simulink model "PAA"  (R2018b)
settings: Solver=FixedStepAuto  StartTime=0.0  StopTime=t_sim  RelTol=1e-3
values from neighbouring files (symbols this model uses):
  FLAG_INPUT_SIGNAL = 0    [PAA_evaluation.m]    (also in door.m)
  noise_gain = 0    [PAA_evaluation.m]    (also in door.m)
  plant_denominator_spr_parallel = [1, -0.1, 0.64]    [PAA_evaluation.m]    (also in door.m)
  t_AdapOff = t_sim+1    (= 4)    [PAA_evaluation.m]    (also in door.m = 5)
  t_AdapOn = 0    [PAA_evaluation.m]    (also in door.m)
  Ts = 0.01    [PAA_evaluation.m]    (also in door.m)
undefined symbols (not defined in the file or in its folder): adap_init
libraries: simulink x3
settings Model: Creator=litingsun  LastModifiedBy=jessl
settings SFSimCC: SimUseLocalCustomCode=off
settings RTWCC: RTWUseLocalCustomCode=off
settings CodeAppCC: StateflowObjectComments=on

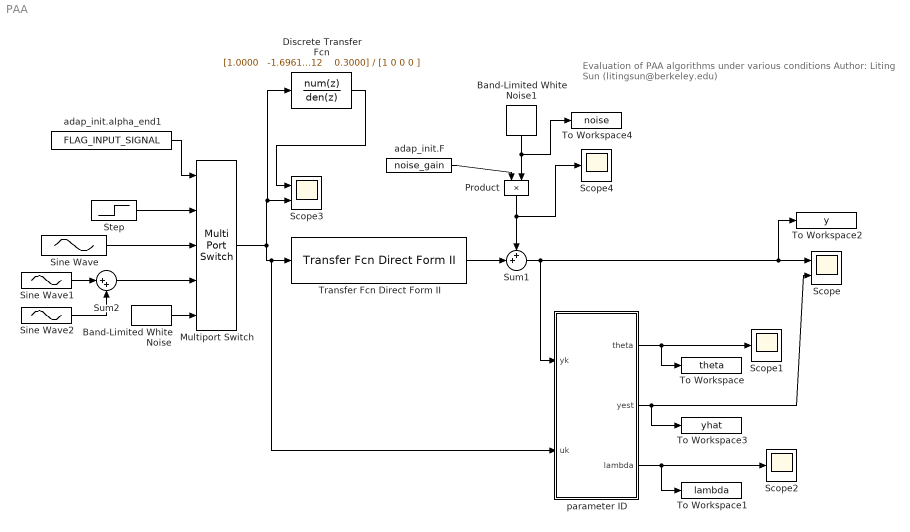
== system PAA ==
  note: Evaluation of PAA algorithms under various conditions
      |
      | Author: Liting Sun (litingsun@berkeley.edu)
  Band-Limited White Noise : simulink/Sources/Band-Limited White Noise  Cov=[0.1]  Ts=Ts  seed=[23341]
  Band-Limited White Noise1 : simulink/Sources/Band-Limited White Noise  Cov=[1]  Ts=Ts  seed=[12345]
  Discrete Transfer Fcn : DiscreteTransferFcn  Numerator="[1.0000   -1.6961    0.4012    0.3000]"  Denominator=[1 0 0 0 ]
  Multiport Switch : MultiPortSwitch  DataPortOrder=Zero-based contiguous  Inputs=4  zeroidx=on
  Product : Product
  Scope : Scope  NumInputPorts=2
  Scope1 : Scope
  Scope2 : Scope
  Scope3 : Scope  NumInputPorts=2
  Scope4 : Scope
  Sine Wave : Sin  Amplitude=0.1  Frequency=2*pi  SampleTime=0
  Sine Wave1 : Sin  Amplitude=1.1  Frequency=10  SampleTime=0
  Sine Wave2 : Sin  Amplitude=2.7  Frequency=97  SampleTime=0
  Step : Step  SampleTime=Ts
  Sum1 : Sum  Inputs=++|
  Sum2 : Sum  Inputs=|++
  To Workspace : ToWorkspace  VariableName=theta  SaveFormat=Structure With Time  SampleTime=-1
  To Workspace1 : ToWorkspace  VariableName=lambda  SaveFormat=Structure With Time  SampleTime=-1
  To Workspace2 : ToWorkspace  VariableName=y  SaveFormat=Structure With Time  SampleTime=-1
  To Workspace3 : ToWorkspace  VariableName=yhat  SaveFormat=Structure With Time  SampleTime=-1
  To Workspace4 : ToWorkspace  VariableName=noise  SaveFormat=Structure With Time  SampleTime=-1
  Transfer Fcn Direct Form II : simulink/Additional Math & Discrete/Additional Discrete/Transfer Fcn Direct Form II  NumCoefVec=[0, 2, 1]  DenCoefVec=plant_denominator_spr_parallel(2:3)  vinit=0.0  RndMeth=Zero  DoSatur=off
      settings: SourceProductName=Simulink  SourceProductBaseCode=SL
  "adap_init.F " : Constant  Value=noise_gain
  adap_init.alpha_end1 : Constant  Value=FLAG_INPUT_SIGNAL
  parameter ID : Subsystem
  wires:
  parameter ID/1(theta) -> Scope1/1, To Workspace/1
  parameter ID/3(lambda) -> Scope2/1, To Workspace1/1
  parameter ID/2(yest) -> Scope/2, To Workspace3/1
  Multiport Switch/1 -> Discrete Transfer Fcn/1, Scope3/2, parameter ID/2(uk), Transfer Fcn Direct Form II/1
  Transfer Fcn Direct Form II/1 -> Sum1/2
  Band-Limited White Noise1/1 -> To Workspace4/1, Product/2
  Product/1 -> Scope4/1, Sum1/1
  "adap_init.F "/1 -> Product/1
  Sum1/1 -> Scope/1, To Workspace2/1, parameter ID/1(yk)
  adap_init.alpha_end1/1 -> Multiport Switch/1
  Step/1 -> Multiport Switch/2
  Band-Limited White Noise/1 -> Multiport Switch/5
  Sine Wave/1 -> Multiport Switch/3
  Sine Wave1/1 -> Sum2/1
  Sine Wave2/1 -> Sum2/2
  Sum2/1 -> Multiport Switch/4
  Discrete Transfer Fcn/1 -> Scope3/1

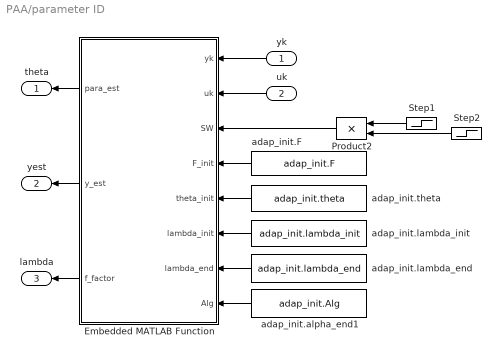
== system PAA/parameter ID ==
  yk : Inport
  uk : Inport  Port=2
  Embedded MATLAB Function : MATLAB Function  TreatAsAtomicUnit=on
  Product2 : Product  RndMeth=Zero
  Step1 : Step  Time=t_AdapOn  SampleTime=Ts
  Step2 : Step  Time=t_AdapOff  Before=1  After=0  SampleTime=Ts
  "adap_init.F " : Constant  Value=adap_init.F
  adap_init.alpha_end1 : Constant  Value=adap_init.Alg
  adap_init.lambda_end : Constant  Value=adap_init.lambda_end
  adap_init.lambda_init : Constant  Value=adap_init.lambda_init
  adap_init.theta : Constant  Value=adap_init.theta
  theta : Outport
  yest : Outport  Port=2
  lambda : Outport  Port=3
  wires:
  uk/1 -> Embedded MATLAB Function/2(uk)
  Embedded MATLAB Function/3(f_factor) -> lambda/1
  "adap_init.F "/1 -> Embedded MATLAB Function/4(F_init)
  adap_init.alpha_end1/1 -> Embedded MATLAB Function/8(Alg)
  Embedded MATLAB Function/1(para_est) -> theta/1
  adap_init.lambda_init/1 -> Embedded MATLAB Function/6(lambda_init)
  yk/1 -> Embedded MATLAB Function/1(yk)
  adap_init.lambda_end/1 -> Embedded MATLAB Function/7(lambda_end)
  Product2/1 -> Embedded MATLAB Function/3(SW)
  Step2/1 -> Product2/2
  Step1/1 -> Product2/1
  adap_init.theta/1 -> Embedded MATLAB Function/5(theta_init)
  Embedded MATLAB Function/2(y_est) -> yest/1

== matlab function PAA/parameter ID/Embedded MATLAB Function ==
  data: yk input; uk input; SW input; para_est output; y_est output; f_factor output; F_init input; theta_init input; lambda_init input; lambda_end input; Alg input
function [para_est, y_est, f_factor] = PAA(yk,uk, SW, F_init,theta_init,lambda_init,lambda_end, Alg) %#eml
persistent N y u phi F theta lambda yhat ehat ykhat ek vk iter phi_F_phi delta_theta;
persistent ykhat_post ek_post flag_series_parallel theta_comp; 
% PAA algorithms implementation for two order systems: 
% two numberator parameters and two denominator parameters
%                 b0+b1*z^-1
% y(k) = ----------------------u(k-1)
%            1+a1*z^-1 +a2*z^-2
% ==> theta = [a1, a2, b0, b1]', phi = [-y(k-1), -y(k-2), u(k-1), u(k-2)]';
% ============================================================
%   Copyright (c) 2015-, Liting Sun, litingsun@berkeley.edu
%   Author(s): Liting Sun
%              University of California at Berkeley
%              Berkeley, CA, 94720, USA
% ============================================================
if isempty(N)
    % initialize all necessary parameters     
    N       = uint16(1);
    y       = zeros(2,1);
    yhat    = zeros(2,1);
    ehat    = zeros(2,1); % store the posterior estimation error
    u       = zeros(2,1);
    phi     = zeros(4,1);
    
    F       = F_init;
    theta   = theta_init; 
    lambda  = lambda_init;
    
    ykhat       = 0;
    ykhat_post  = 0;
    ek          = 0;
    ek_post     = 0;
    
    iter        = 0;
    phi_F_phi   = 0;
    delta_theta = 0*theta_init;
    
    flag_series_parallel = 1;
    theta_comp  = theta;
    
end
if SW == 0
    %========= Adaptation turned off. ==========
    % update observation vector
    ykhat     = [-yhat(1), -yhat(2), u(1), u(2)]*theta;
    
    y(2)     = y(1);
    y(1)     = yk;
    u(2)     = u(1);
    u(1)     = uk;
    yhat(2)  = yhat(1);
    yhat(1)  = yk;
    
    para_est = theta;
    f_factor = lambda;
    y_est    = ykhat;
    
    
else
    switch(Alg)
        case 0 % series-parallel structure
            %% read data
            phi = [-y(1), -y(2), u(1), u(2)]';
            % a priori estimate
            ykhat = phi'*theta;
            % a priori estimation error
            ek = yk - ykhat;
            phi_F_phi = phi'*F*phi;
            delta_theta = (F*phi*ek/(1+phi_F_phi));
            % parameter estimation update
            theta = theta + delta_theta;
            % adaptation gain update
            F = 1/lambda * ( F - F*(phi*phi')*F / (lambda+phi_F_phi) );
            % a posteriori prediction
            ykhat_post = phi'*theta;
            ek_post = yk - ykhat_post;
            % update the forgetting factor
            lambda = lambda_end - (lambda_end-lambda) * 0.98;
            % update observation vector
            y(2)     = y(1);
            y(1)     = yk;
            u(2)     = u(1);
            u(1)     = uk;
            
        case 1     % parallel structure
            %% read data
            phi = [-yhat(1), -yhat(2), u(1), u(2)]';
            % a priori estimation 
            ykhat = phi'*theta;
            % a priori estimation error
            ek = yk - ykhat;
            phi_F_phi = phi'*F*phi;
            % parameter estimation update
            delta_theta = (F*phi*ek/(1+phi_F_phi));
            theta = theta + delta_theta;
            F = 1/lambda * ( F - F*(phi*phi')*F / (lambda+phi_F_phi) );
            % a posteriori prediction
            ykhat_post = phi'*theta;
            ek_post = yk - ykhat_post;
            lambda = lambda_end - (lambda_end-lambda) * 0.98;
            % update observation vector
            u(2)     = u(1);
            u(1)     = uk;
            yhat(2) = yhat(1);
            yhat(1) = ykhat_post;
        case 2      
            % parallel structure with a fixed compensator and the fixed compensator comes from sp-PAA
            % i.e, we are using two-stage PAA
            %% first stage: sp PAA for a rough estimation
            if flag_series_parallel == 1
                % read data
                phi = [-y(1), -y(2), u(1), u(2)]';
                % a priori estimate
                ykhat = phi'*theta;
                % a priori estimation error
                ek = yk - ykhat;
                phi_F_phi = phi'*F*phi;
                delta_theta = (F*phi*ek/(1+phi_F_phi));
                % parameter estimation update
                theta = theta + delta_theta;
                % adaptation gain update
                F = 1/lambda * ( F - F*(phi*phi')*F / (lambda+phi_F_phi) );
                % a posteriori prediction
                ykhat_post = phi'*theta;
                ek_post = yk - ykhat_post;
                % update the forgetting factor
                lambda = lambda_end - (lambda_end-lambda) * 0.98;
                % update observation vector
                y(2)     = y(1);
                y(1)     = yk;
                u(2)     = u(1);
                u(1)     = uk;
                yhat(2)  = yhat(1);
                yhat(1)  = yk;
                ehat(2)  = ehat(1);
                ehat(1)  = ek_post;
                if iter >= 300 % terminate the sp PAA after a fixed number of iterations
                    % set the flag to zero
                    flag_series_parallel = 0;
                    % reset the adaptation gain. It does not necessarily be
                    % F_init, and you are free to set it other values. The
                    % goal here is to make the adaptation gain large enough
                    % so that the second stage is effective.
                    F = F_init;
                    % set the current theta as the compensator coefficients
                    theta_comp = theta;
                end
            else
                % read data
                phi = [-yhat(1), -yhat(2), u(1), u(2)]';
                % a priori estimation 
                ykhat = phi'*theta;
                % a priori estimation error
                ek = yk - ykhat;
                phi_F_phi = phi'*F*phi;
                vk = ek + theta_comp(1)*ehat(1)+theta_comp(2)*ehat(2);
                % parameter estimation update
                delta_theta = (F*phi*vk/(1+phi_F_phi));
                theta = theta + delta_theta;
                F = 1/lambda * ( F - F*(phi*phi')*F / (lambda+phi_F_phi) );
                % a posteriori prediction
                ykhat_post = phi'*theta;
                ek_post = yk - ykhat_post;
                lambda = lambda_end - (lambda_end-lambda) * 0.98;
                % update observation vector
                u(2)     = u(1);
                u(1)     = uk;
                yhat(2) = yhat(1);
                yhat(1) = ykhat_post;
                ehat(2)  = ehat(1);
                ehat(1)  = ek_post;
            end
            
    end
    
    iter = iter + 1; % iteration update
    % +++++++++++++++++++++++++++++++++++++++++++
    para_est = theta;
    f_factor = lambda;
    y_est    = ykhat_post;
end
